simulink model "erics_testing_file"  (R2025b)
settings: Solver=VariableStepAuto  StartTime=0.0  StopTime=10.0  RelTol=1e-3
undefined symbols (not defined in the file or in its folder): constantsSTADPOLE
settings Model: Creator=Eric  LastModifiedBy=Eric

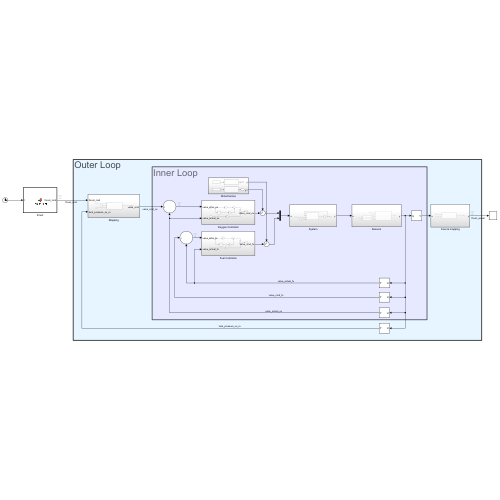
[thumbnail: Simulink's stored preview of the top-level diagram]
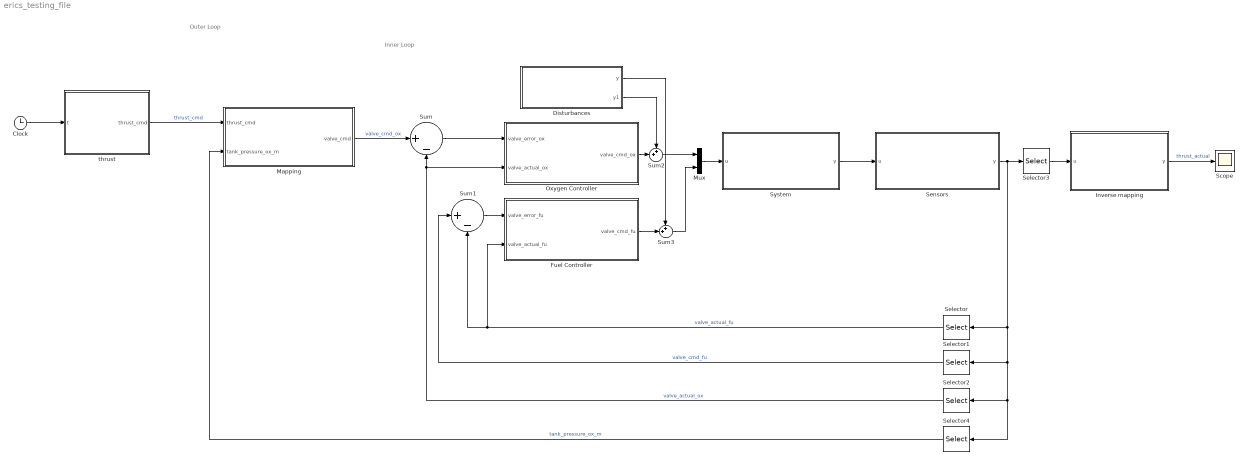
== system erics_testing_file ==
  note: Outer Loop
  note: Inner Loop
  Clock : Clock
  Disturbances : Subsystem
  Fuel Controller : Subsystem
  Inverse mapping : Subsystem
  Mapping : Subsystem
  Mux : Mux  Inputs=2
  Oxygen Controller : Subsystem
  Scope : Scope
      settings: ActiveDisplayYMinimum=-7502.6873499381991  ActiveDisplayYMaximum=6603.0465568308964
  Selector : Selector  InputPortWidth=6  IndexOptions=Index vector (dialog)  Indices=4  OutputSizes=1
  Selector1 : Selector  InputPortWidth=6  IndexOptions=Index vector (dialog)  Indices=3  OutputSizes=1
  Selector2 : Selector  InputPortWidth=6  IndexOptions=Index vector (dialog)  Indices=2  OutputSizes=1
  Selector3 : Selector  InputPortWidth=6  IndexOptions=Index vector (dialog)  Indices=1  OutputSizes=1
  Selector4 : Selector  InputPortWidth=6  IndexOptions=Index vector (dialog)  Indices=5  OutputSizes=1
  Sensors : Subsystem
  Sum : Sum  Inputs=|+-
  Sum1 : Sum  Inputs=|+-
  Sum2 : Sum  Inputs=++|
  Sum3 : Sum  Inputs=++|
  System : Subsystem
  thrust : MATLAB Function  TreatAsAtomicUnit=on
  wires:
  Clock/1 -> thrust/1(t)
  Inverse mapping/1(y) -> Scope/1  "thrust_actual"
  thrust/1(thrust_cmd) -> Mapping/1(thrust_cmd)  "thrust_cmd"
  Sum/1 -> Oxygen Controller/1(valve_error_ox)
  Mapping/1(valve_cmd) -> Sum/1  "valve_cmd_ox"
  Oxygen Controller/1(valve_cmd_ox) -> Sum2/2
  System/1(y) -> Sensors/1(u)
  Sensors/1(y) -> Selector4/1, Selector2/1, Selector1/1, Selector/1, Selector3/1
  Sum1/1 -> Fuel Controller/1(valve_error_fu)
  Mux/1 -> System/1(u)
  Fuel Controller/1(valve_cmd_fu) -> Sum3/2
  Selector/1 -> Fuel Controller/2(valve_actual_fu), Sum1/2  "valve_actual_fu"
  Selector1/1 -> Sum1/1  "valve_cmd_fu"
  Selector2/1 -> Oxygen Controller/2(valve_actual_ox), Sum/2  "valve_actual_ox"
  Selector3/1 -> Inverse mapping/1(u)
  Sum2/1 -> Mux/1
  Disturbances/2(y1) -> Sum2/1
  Disturbances/1(y) -> Sum3/1
  Sum3/1 -> Mux/2
  Selector4/1 -> Mapping/2(tank_pressure_ox_m)  "tank_pressure_ox_m"

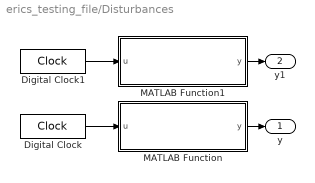
== system erics_testing_file/Disturbances ==
  Digital Clock : DigitalClock
  Digital Clock1 : DigitalClock
  MATLAB Function : MATLAB Function  TreatAsAtomicUnit=on
  MATLAB Function1 : MATLAB Function  TreatAsAtomicUnit=on
  y : Outport
  y1 : Outport  Port=2
  wires:
  MATLAB Function/1(y) -> y/1
  Digital Clock/1 -> MATLAB Function/1(u)
  MATLAB Function1/1(y) -> y1/1
  Digital Clock1/1 -> MATLAB Function1/1(u)

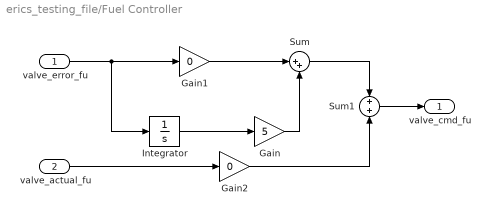
== system erics_testing_file/Fuel Controller ==
  valve_error_fu : Inport
  valve_actual_fu : Inport  Port=2
  Gain : Gain  Gain=5
  Gain1 : Gain  Gain=0
  Gain2 : Gain  Gain=0
  Integrator : Integrator
  Sum : Sum  Inputs=|++
  Sum1 : Sum  Inputs=+|+
  valve_cmd_fu : Outport
  wires:
  valve_error_fu/1 -> Integrator/1, Gain1/1
  Integrator/1 -> Gain/1
  Gain/1 -> Sum/2
  Sum/1 -> Sum1/1
  Gain1/1 -> Sum/1
  Sum1/1 -> valve_cmd_fu/1
  valve_actual_fu/1 -> Gain2/1
  Gain2/1 -> Sum1/2

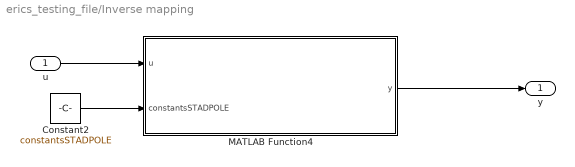
== system erics_testing_file/Inverse mapping ==
  u : Inport
  Constant2 : Constant  Value=constantsSTADPOLE  OutDataTypeStr=Bus: slBus1
  MATLAB Function4 : MATLAB Function  TreatAsAtomicUnit=on
  y : Outport
  wires:
  MATLAB Function4/1(y) -> y/1
  u/1 -> MATLAB Function4/1(u)
  Constant2/1 -> MATLAB Function4/2(constantsSTADPOLE)

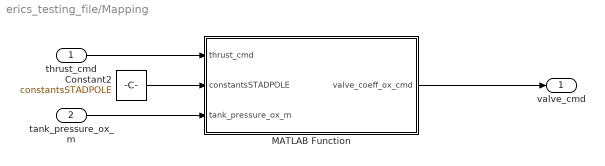
== system erics_testing_file/Mapping ==
  thrust_cmd : Inport
  tank_pressure_ox_m : Inport  Port=2
  Constant2 : Constant  Value=constantsSTADPOLE  OutDataTypeStr=Bus: slBus1
  MATLAB Function : MATLAB Function  TreatAsAtomicUnit=on
  valve_cmd : Outport
  wires:
  MATLAB Function/1(valve_coeff_ox_cmd) -> valve_cmd/1
  thrust_cmd/1 -> MATLAB Function/1(thrust_cmd)
  Constant2/1 -> MATLAB Function/2(constantsSTADPOLE)
  tank_pressure_ox_m/1 -> MATLAB Function/3(tank_pressure_ox_m)

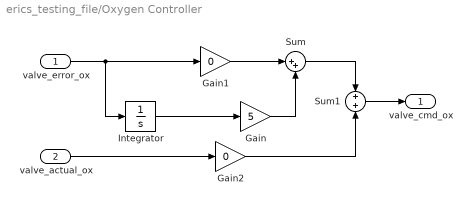
== system erics_testing_file/Oxygen Controller ==
  valve_error_ox : Inport
  valve_actual_ox : Inport  Port=2
  Gain : Gain  Gain=5
  Gain1 : Gain  Gain=0
  Gain2 : Gain  Gain=0
  Integrator : Integrator
  Sum : Sum  Inputs=|++
  Sum1 : Sum  Inputs=+|+
  valve_cmd_ox : Outport
  wires:
  valve_error_ox/1 -> Gain1/1, Integrator/1
  Integrator/1 -> Gain/1
  Gain1/1 -> Sum/1
  Gain/1 -> Sum/2
  Sum/1 -> Sum1/1
  valve_actual_ox/1 -> Gain2/1
  Sum1/1 -> valve_cmd_ox/1
  Gain2/1 -> Sum1/2

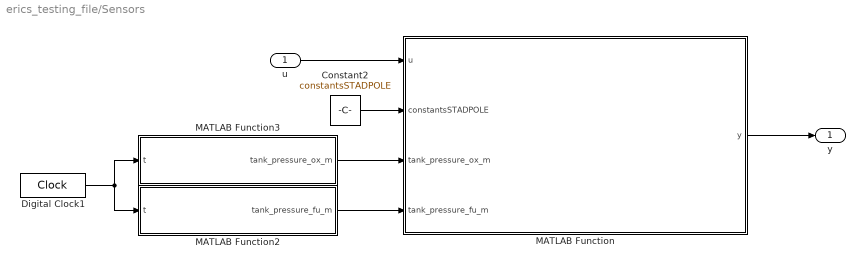
== system erics_testing_file/Sensors ==
  u : Inport
  Constant2 : Constant  Value=constantsSTADPOLE  OutDataTypeStr=Bus: slBus1
  Digital Clock1 : DigitalClock
  MATLAB Function : MATLAB Function  TreatAsAtomicUnit=on
  MATLAB Function2 : MATLAB Function  TreatAsAtomicUnit=on
  MATLAB Function3 : MATLAB Function  TreatAsAtomicUnit=on
  y : Outport
  wires:
  MATLAB Function/1(y) -> y/1
  u/1 -> MATLAB Function/1(u)
  Constant2/1 -> MATLAB Function/2(constantsSTADPOLE)
  MATLAB Function3/1(tank_pressure_ox_m) -> MATLAB Function/3(tank_pressure_ox_m)
  Digital Clock1/1 -> MATLAB Function3/1(t), MATLAB Function2/1(t)
  MATLAB Function2/1(tank_pressure_fu_m) -> MATLAB Function/4(tank_pressure_fu_m)

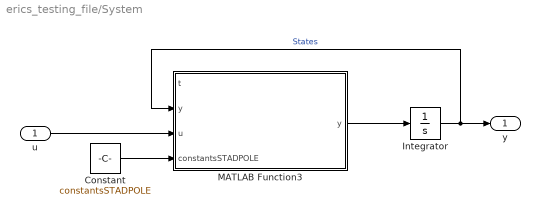
== system erics_testing_file/System ==
  u : Inport
  Constant : Constant  Value=constantsSTADPOLE  OutDataTypeStr=Bus: slBus1
  Integrator : Integrator  InitialCondition=constantsSTADPOLE.init_cond
  MATLAB Function3 : MATLAB Function  TreatAsAtomicUnit=on
  y : Outport
  wires:
  MATLAB Function3/1(y) -> Integrator/1
  u/1 -> MATLAB Function3/3(u)
  Integrator/1 -> MATLAB Function3/2("y "), y/1  "States"
  Constant/1 -> MATLAB Function3/4(constantsSTADPOLE)

== matlab function erics_testing_file/Mapping/MATLAB Function ==
  data: thrust_cmd input; valve_coeff_ox_cmd output; constantsSTADPOLE input; tank_pressure_ox_m input
function valve_coeff_ox_cmd = thrust_to_valve_mapping(thrust_cmd, constantsSTADPOLE, tank_pressure_ox_m)

throat_area = constantsSTADPOLE.a_t;                % [m^2]
thrust_coeff = constantsSTADPOLE.c_f;               % [unitless]
char_vel = constantsSTADPOLE.c_star;                % [m/s]
of_ratio = constantsSTADPOLE.OF_target;             % [unitless]
rho_ox = constantsSTADPOLE.dens_o;                  % [kg/m^3]
discharge_coeff_ox = constantsSTADPOLE.d_coeff_ox;  % [unitless],  -------------Random value just to get the code to run
orifice_area_ox = constantsSTADPOLE.a_i_o;          % [m^2],  -------------Random value just to get the code to run
rho_water = constantsSTADPOLE.dens_w;               % [kg/m^3]

% Valve Coefficient Calculations 
chamber_pressure_cmd = thrust_cmd / (throat_area * thrust_coeff);   % [Pa]
massflow_tot_cmd = chamber_pressure_cmd * throat_area / char_vel;   % [kg/s]
massflow_ox_cmd = massflow_tot_cmd * of_ratio / (of_ratio + 1);     % [kg/s]
friction_pressure_drop_ox = 96402.2 * massflow_ox_cmd^2;
injector_pressure_ox_cmd = chamber_pressure_cmd + (massflow_ox_cmd ^ 2) / (2 * rho_ox * (discharge_coeff_ox * orifice_area_ox) ^ 2); % [Pa]
valve_coeff_ox_cmd = massflow_ox_cmd * sqrt(max(1 / (rho_ox * rho_water * (tank_pressure_ox_m - friction_pressure_drop_ox - injector_pressure_ox_cmd)), 0)); % [m^3.5/kg^0.5]

% NEED VALVE COEFFICIENT TO VALVE ANGLE FUNCTION

== matlab function erics_testing_file/thrust ==
  data: t input; thrust_cmd output
function thrust_cmd = ThrustPlant(t)
% %THRUSTPLANT 
% %   random plant function for the thrust in the engine
% if t < 2
%     thrust_cmd = 0; %[N]
% elseif mod(t,5) < 3
%     thrust_cmd = 1500;
% else
%     thrust_cmd = 1500 - 500 * sin(mod(t,5) * pi / 2);
% 
% end
% %cosint(t*pi/180);

%thrust_cmd = 1500;
if t < 3.0
    thrust_cmd = 1000; % [N] Step 1: 0s to 3s
elseif t < 6.0
    thrust_cmd = 1500; % [N] Step 2: 3s to 6s
else
    thrust_cmd = 1000;    % [N] Step 3: 6s to 10s
end

end

== matlab function erics_testing_file/Sensors/MATLAB Function3 ==
  data: t input; tank_pressure_ox_m output
function tank_pressure_ox_m = oxygen_tank_pressure(t)

% Simulate oxygen tank pressure, for now, assume constant at 550 psi or 
% 3.792 MPa

tank_pressure_ox_m = 3.792E6; % [Pa]

== matlab function erics_testing_file/Sensors/MATLAB Function2 ==
  data: t input; tank_pressure_fu_m output
function tank_pressure_fu_m = fuel_tank_pressure(t)

% Simulate fuel tank pressure, for now, assume constant at 550 psi or 3.792
% MPa

tank_pressure_fu_m = 3.792E6; % [MPa]

== matlab function erics_testing_file/System/MATLAB Function3 ==
  data: t input; y input; u input; y output; constantsSTADPOLE input
function y = system_model(t, y, u, constantsSTADPOLE)
    
    % y(1)' = time rate of mass flow oxygen [kg/s^2]
    % y(2)' = time rate of mass flow fuel [kg/s^2]
    % y(3)' = time rate of chamber pressure [Pa/s]
    % y(4)' = time rate of oxygen injector press [Pa/s]
    % y(5)' = time rate of fuel injector press [Pa/s]
    % y(6)' = time rate of oxygen pressure at valve [Pa/s]
    % y(7)' = time rate of fuel pressure at valve [Pa/s]

    % y(1) = mass flow oxygen across pipe [kg/s]
    % y(2) = mass flow fuel across pipe [kg/s]
    % y(3) = chamber pressure [Pa]
    % y(4) = oxygen pressure at inj [Pa]
    % y(5) = fuel pressure at inj [Pa]
    % y(6) = oxygen pressure at valve [Pa]
    % y(7) = fuel pressure at valve [Pa]
    
    a_t= constantsSTADPOLE.a_t ; % [m^2], throat area
    
    dens_o = constantsSTADPOLE.dens_o; % [kg/m^3], liquid oxygen density, at 90 K and 1 atm
    dens_f = constantsSTADPOLE.dens_f ; % [kg/m^3], fuel density, at 293 K and 1 atm
    dens_w = constantsSTADPOLE.dens_w ; % [kg/m^3], water density
    g = constantsSTADPOLE.g ; % [m/s^2], acceleration due to gravity
    a_i_o = constantsSTADPOLE.a_i_o; % [m^2] area injector ox
    a_i_f = constantsSTADPOLE.a_i_f ; % [m^2] area injector fuel
    r = constantsSTADPOLE.r ; % [J/kg-K], specific gas constant of exhaust (molecular weight 18.8 g/mol)
    c_star = constantsSTADPOLE.c_star ; % [m/s] characteristic velocity
    of = constantsSTADPOLE.OF_target;

    c_fric = 0.03; % [unitless], line friction coefficient
    c_d_o = constantsSTADPOLE.d_coeff_ox; % [unitless], oxygen injector coefficient
    c_d_f = constantsSTADPOLE.d_coeff_fu; % [unitless], fuel injector coefficient
    l_eq_o = 7 * 0.0254; % [m], oxygen equivalent line length 
    l_eq_f = 7 * 0.0254; % [m], fuel equivalent line length 
    l_o = 120 * 0.0254; % [m], oxygen line length
    l_f = 60 * 0.0254; % [m], fuel line length
    d = (0.5 - 2 * 0.065) * 0.0254; % [m], line diameter
    v_c = 1.103170594 * 1e-3; % [m^3], chamber volume
    a_l = pi * (d / 2) ^ 2; % [m^2], line area
  
    v_l_o = a_l * l_o;
    v_l_f = a_l * l_f;
    t_o = 90; 
    t_f = 293;

    % Assume constant?
    c_v_o = u(1,1); %AngleToCoefficient(u(1,1));  % 1.231e-06; [m^3.5/kg^0.5], oxygen valve coefficient
    c_v_f = u(2,1); %AngleToCoefficient(u(2,1));  % 1.231e-06; [], fuel valve coefficient
    p_tank_o = 3.792E6; % [Pa]
    p_tank_f = 3.792E6; % [Pa]
    t_c = 3570; % [K], chamber temperature
    

    del_p_i_o = 1 / (2 * dens_o * (c_d_o * a_i_o) ^ 2); 
    del_p_l_o = 96402.2;
    del_p_i_f = 1 / (2 * dens_f * (c_d_f * a_i_f) ^ 2); 
    del_p_l_f = 2082581.1;
    

    % Momentum equations
    % massflow across pipe
    % mdot_pipe_ox = (y(4) - y(3) - del_p_l_o * y(1) * sqrt(y(1)^2 + 1e-6)) * a_l / l_o;
    % mdot_pipe_fu = (y(5) - y(3) - del_p_l_f * y(2) * sqrt(y(2)^2 + 1e-6)) * a_l / l_f;
    mddot_pipe_ox = (y(6) - y(4) - del_p_l_o * y(1) * sqrt(y(1)^2 + 1e-6)) * a_l / l_o;
    mddot_pipe_fu = (y(7) - y(5) - del_p_l_f * y(2) * sqrt(y(2)^2 + 1e-6)) * a_l / l_f;

    % Valve massflows
    ValveOX = dens_o * dens_w * (p_tank_o - y(6));
    ValveFU = dens_f * dens_w * (p_tank_f - y(7));
    mdot_valve_ox = c_v_o * ValveOX / sqrt(abs(ValveOX) + 1e2);
    mdot_valve_fu = c_v_f * ValveFU / sqrt(abs(ValveFU) + 1e2);

    % Injector massflows
    InjectorOX = 2 * dens_o *(y(4)-y(3));
    InjectorFU = 2 * dens_f * (y(5)-y(3));
    mdot_inj_ox = c_d_o * a_i_o * InjectorOX / sqrt(abs(InjectorOX)+1e2);
    mdot_inj_fu = c_d_f * a_i_f * InjectorFU / sqrt(abs(InjectorFU)+1e2);

    % Pressure at the end of the valve
    valve_ox_dot = 1e9 / (v_l_o * dens_o) * (mdot_valve_ox - y(1));
    valve_fu_dot = 1e9 / (v_l_f * dens_f) * (mdot_valve_fu - y(2));

    inj_ox_dot = 1e9 / (v_l_o*dens_o) * (y(1) - mdot_inj_ox);
    inj_fu_dot = 1e9 / (v_l_f*dens_f) * (y(2) - mdot_inj_fu);

    % Chamber Pressure equations
    pdot_chamber = (r * t_c / v_c) * (mdot_inj_ox + mdot_inj_fu - a_t * y(3) / c_star);

    % Final system
    y = [mddot_pipe_ox; mddot_pipe_fu; pdot_chamber; inj_ox_dot; inj_fu_dot; valve_ox_dot; valve_fu_dot];
end

== matlab function erics_testing_file/Inverse mapping/MATLAB Function4 ==
  data: u input; y output; constantsSTADPOLE input
function y = valve_to_thrust_mapping(u, constantsSTADPOLE)

throat_area = constantsSTADPOLE.a_t; % [m^2]
thrust_coeff = constantsSTADPOLE.c_f; % [unitless]

y = u * thrust_coeff * throat_area;

== matlab function erics_testing_file/Sensors/MATLAB Function ==
  data: u input; y output; constantsSTADPOLE input; tank_pressure_ox_m input; tank_pressure_fu_m input
function y = sensor_function(u, constantsSTADPOLE, tank_pressure_ox_m, tank_pressure_fu_m)

% *************************************************************************
% Constants

of_ratio = constantsSTADPOLE.OF_target; % [unitless]
rho_ox = constantsSTADPOLE.dens_o; % [kg/m^3]
rho_fu = constantsSTADPOLE.dens_f; % [kg/m^3]
discharge_coeff_ox = constantsSTADPOLE.d_coeff_ox; % [unitless],  -------------Random value just to get the code to run
discharge_coeff_fu = constantsSTADPOLE.d_coeff_fu; % [unitless],  -------------Random value just to get the code to run
orifice_area_ox = constantsSTADPOLE.a_i_o; % [m^2],  -------------Random value just to get the code to run
orifice_area_fu = constantsSTADPOLE.a_i_f; % [m^2],  -------------Random value just to get the code to run
throat_area = constantsSTADPOLE.a_t; % [m^2]
char_vel = constantsSTADPOLE.c_star; % [m/s]

% 150 psi at max thrust, quarter at 50%
rho_water = constantsSTADPOLE.dens_w; % [kg/m^3]

% *************************************************************************
% Inputs

% u(1) = mass flow oxygen across pipe [kg/s]
% u(2) = mass flow fuel across pipe [kg/s]
% u(3) = chamber pressure [Pa]
% u(4) = oxygen pressure at inj [Pa]
% u(5) = fuel pressure at inj [Pa]
% u(6) = oxygen pressure at valve [Pa]
% u(7) = fuel pressure at valve [Pa]

chamber_pressure_m = u(3);
injector_pressure_ox_m = u(4);
injector_pressure_fu_m = u(5);

% *************************************************************************
% Fuel Valve command

% Calculates fuel valve command based on oxygen injector pressure and
% chamber pressure

% Valve coefficient equations
delta_p_injector_ox_calc = max(injector_pressure_ox_m - chamber_pressure_m, 0); % [Pa]
term_1 = sqrt(2 * delta_p_injector_ox_calc * rho_ox); % [kg/m^2-s]
massflow_ox_calc = discharge_coeff_ox * orifice_area_ox * term_1; % [kg/s]
massflow_fu_calc = massflow_ox_calc / of_ratio; % [kg/s]
injector_pressure_fu_calc = chamber_pressure_m + (massflow_fu_calc ^ 2) / (2 * rho_fu * (discharge_coeff_fu * orifice_area_fu) ^ 2); % [Pa]
friction_pressure_drop_fu = massflow_fu_calc^2 * 2082581.1;
valve_coeff_fu_cmd = massflow_fu_calc *  sqrt(max(1 / (rho_fu * rho_water * (tank_pressure_fu_m - friction_pressure_drop_fu - injector_pressure_fu_calc)), 0)); % [m^3.5/kg^0.5]

% NEED COEFFICIENT TO ANGLE MAPPING

% *************************************************************************
% Fuel Valve actual

delta_p_injector_fu_calc = max(injector_pressure_fu_m - chamber_pressure_m, 0); % [Pa]
term_2 = sqrt(2 * delta_p_injector_fu_calc * rho_fu); % [kg/m^2-s]
massflow_fu_calc2 = discharge_coeff_fu * orifice_area_fu * term_2; % [kg/s]
valve_coeff_fu_actual = massflow_fu_calc2 *  sqrt(max(1 / (rho_fu * rho_water * (tank_pressure_fu_m - friction_pressure_drop_fu - injector_pressure_fu_m)), 0)); % [m^3.5/kg^0.5]

% *************************************************************************
% Oxygen Valve actual

% massflow_tot_m = chamber_pressure_m * throat_area / char_vel; % [kg/s]
% massflow_ox_m = massflow_tot_m * of_ratio / (of_ratio + 1); % [kg/s]
friction_pressure_drop_ox = 96402.2 * massflow_ox_calc^2;
valve_coeff_ox_actual = massflow_ox_calc * sqrt(max(1 / (rho_ox * rho_water * (tank_pressure_ox_m - friction_pressure_drop_ox - injector_pressure_ox_m)), 0)); % [m^3.5/kg^0.5]

% *************************************************************************
% Outputs

y = [chamber_pressure_m; valve_coeff_ox_actual; valve_coeff_fu_cmd; valve_coeff_fu_actual; tank_pressure_ox_m; tank_pressure_fu_m];

== matlab function erics_testing_file/Disturbances/MATLAB Function ==
  data: u input; y output
function y = valve_disturbance_ox(u)

y = 0;

== matlab function erics_testing_file/Disturbances/MATLAB Function1 ==
  data: u input; y output
function y = valve_disturbance_fu(u)

y = 0;
